simulink model "compare_simulation_modes"  (R2014a)
settings: Solver=ode23tb  SolverMode=SingleTasking  StartTime=0.0  StopTime=0.3  RelTol=1e-4
StartFcn:
  | tic;
StopFcn:
  | toc;
libraries: powerlib x15
Description:
  | Copyright 2008-2014 The MathWorks, Inc.
settings Model: ExtModeTrigMode=oneshot  ExtModeArmWhenConnect=off  ExtModeAutoUpdateStatusClock=off  Creator=MathWorks  LastModifiedBy=cosorio
settings SolverCC: ZeroCrossAlgorithm=Adaptive
settings DataIOCC: LimitDataPoints=off  SaveOutput=off  SaveTime=off  SignalLoggingName=sigsOut
settings OptimizationCC: BlockReduction=off  BooleanDataType=off  ExpressionDepthLimit=2147483647  InitFltsAndDblsToZero=on  EfficientMapNaN2IntZero=off
settings DebuggingCC: SaveWithParameterizedLinksMsg=none  UnderspecifiedInitializationDetection=Classic  CheckExecutionContextPreStartOutputMsg=on  CheckExecutionContextRuntimeOutputMsg=on  SignalResolutionControl=TryResolveAllWithWarning  SolverPrmCheckMsg=none  MultiTaskDSMMsg=warning  MultiTaskCondExecSysMsg=none  SigSpecEnsureSampleTimeMsg=none  FcnCallInpInsideContextMsg=UseLocalSettings  StateNameClashWarn=warning
settings HardwareCC: TargetUnknown=on
settings RTWCC: IncludeERTFirstTime=on
settings GRTTargetCC: TargetFcnLib=ansi_tfl_tmw.mat  CombineOutputUpdateFcns=off  GRTInterface=on

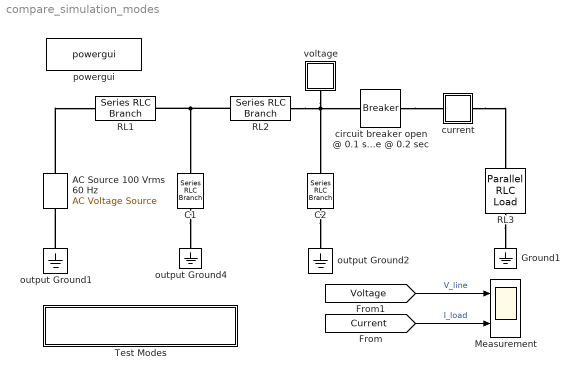
== system compare_simulation_modes ==
  AC Source 100 Vrms 60 Hz : powerlib/Electrical Sources/AC Voltage Source  Description=source block  Amplitude=100*sqrt(2)  Phase=90  Frequency=60  SampleTime=0  Measurements=None
      settings: AttributesFormatString=\n
  C1 : powerlib/Elements/Series RLC Branch  LConnTagsString=__new0  RConnTagsString=__new0  BranchType=C  Resistance=[]  Inductance=[]  SetiL0=off  InitialCurrent=0  Capacitance=0.967e-06  Setx0=off  InitialVoltage=0  Measurements=None
  C2 : powerlib/Elements/Series RLC Branch  LConnTagsString=__new0  RConnTagsString=__new0  BranchType=C  Resistance=[]  Inductance=[]  SetiL0=off  InitialCurrent=0  Capacitance=0.967e-06  Setx0=off  InitialVoltage=0  Measurements=None
  Ground1 : powerlib/Elements/Ground  LConnTagsString=a
  Measurement : Scope  NumInputPorts=2
      settings: YMin=-200~-1  YMax=200~1  SaveName=VI_Data
  RL1 : powerlib/Elements/Series RLC Branch  LConnTagsString=__new0  RConnTagsString=__new0  BranchType=RL  Resistance=2.645  Inductance=70.2e-03  SetiL0=off  InitialCurrent=0  Capacitance=[]  Setx0=off  InitialVoltage=0  Measurements=None
  RL2 : powerlib/Elements/Series RLC Branch  LConnTagsString=__new0  RConnTagsString=__new0  BranchType=RL  Resistance=5.2  Inductance=138e-3  SetiL0=off  InitialCurrent=0  Capacitance=[]  Setx0=off  InitialVoltage=0  Measurements=None
  RL3 : powerlib/Elements/Parallel RLC Load  LConnTagsString=a  RConnTagsString=__new0  NominalVoltage=132.8e3  NominalFrequency=60  ActivePower=75e6  InductivePower=20e6  CapacitivePower=0  Setx0=off  InitialVoltage=0  SetiL0=off  InitialCurrent=0  Measurements=None
      settings: AttributesFormatString=\n
  Test Modes : Subsystem
      settings: OpenFcn=test_simulation_modes
      mask Display: disp('Double click here to\ncompare simulation modes');
  circuit breaker open @ 0.1 sec close @ 0.2 sec : powerlib/Elements/Breaker  InitialState=1  SwitchingTimes="[6/60  12/60]"  External=off  BreakerResistance=0.01  SnubberResistance=inf  SnubberCapacitance=0  Measurements=None  MoreParameters=off  NoBreakLoop=off
      settings: AttributesFormatString=\n
  current : Subsystem
      mask Display: disp('i');
  output Ground1 : powerlib/Elements/Ground  LConnTagsString=a
  output Ground2 : powerlib/Elements/Ground  LConnTagsString=a
  output Ground4 : powerlib/Elements/Ground  LConnTagsString=a
  powergui : powerlib/powergui  Priority=2  SimulationMode=Continuous  SolverType=Tustin  SampleTime=1e-4  frequency=60  SPID=off  DisableSnubberDevices=off  DisableRonSwitches=off  DisableVfSwitches=off  SwTol=0  Interpol=off  DisplayEquations=off  Ts=0  methode=off  frequencyindice=60  Pbase=100e6  ErrMax=1e-4  Iterations=50  UnitsV=kV  UnitsW=MW  FunctionMessages=off  echomessages=off  HookPort=off  EnableUseOfTLC=off  x0status=blocks  RestoreLinks=warning  ResistiveCurrentMeasurement=off  Frange=logspace(0,3,50)  Ylog=off  Xlog=off  ShowGrid=off  save=off  variable=ZData  structure=0  ZoomFFT=on  StartTime=0.0  cycles=1  DisplayStyle=off  fundamental=60  FreqAxis=off  MaxFrequency=1000  frequencyindicesteady=1  RmsSteady=1  display=off
  voltage : Subsystem
      mask Display: disp('v');
  wires:
  [Voltage] -> Measurement/1  "V_line"
  [Current] -> Measurement/2  "I_load"
  connections:
  RL3/RConn1 -- Ground1/LConn1
  AC Source 100 Vrms 60 Hz/RConn1 -- RL1/LConn1
  output Ground1/LConn1 -- AC Source 100 Vrms 60 Hz/LConn1
  RL2/LConn1 -- RL1/RConn1 -- C1/LConn1
  C1/RConn1 -- output Ground4/LConn1
  C2/RConn1 -- output Ground2/LConn1
  RL2/RConn1 -- circuit breaker open @ 0.1 sec close @ 0.2 sec/LConn1 -- voltage/RConn1 -- C2/LConn1
  circuit breaker open @ 0.1 sec close @ 0.2 sec/RConn1 -- current/LConn1
  current/RConn1 -- RL3/LConn1

== system compare_simulation_modes/Test Modes ==

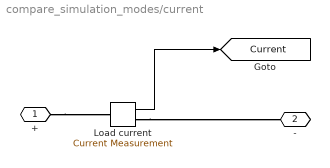
== system compare_simulation_modes/current ==
  Load current : powerlib/Measurements/Current Measurement  Tag=PoWeRsYsTeMmEaSuReMeNt  PhasorSimulation=off  OutputType=Magnitude  PSBequivalent=0
  + : PMIOPort  Port=1  Side=Left
  - : PMIOPort  Port=2  Side=Right
  tag scope: Current=global
  wires:
  Load current/1 -> [Current]
  connections:
  +/RConn1 -- Load current/LConn1
  Load current/RConn1 -- -/RConn1

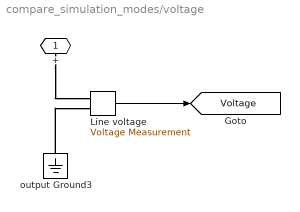
== system compare_simulation_modes/voltage ==
  Line voltage : powerlib/Measurements/Voltage Measurement  Tag=PoWeRsYsTeMmEaSuReMeNt  PhasorSimulation=off  OutputType=Magnitude  PSBequivalent=0
  output Ground3 : powerlib/Elements/Ground  LConnTagsString=a
  + : PMIOPort  Port=1  Side=Right
  tag scope: Voltage=global
  wires:
  Line voltage/1 -> [Voltage]
  connections:
  output Ground3/LConn1 -- Line voltage/LConn2
  +/RConn1 -- Line voltage/LConn1
